simulink model "models_lib"  (R2016a)
settings: Solver=FixedStepAuto  StartTime=0.0  StopTime=30  FixedStep=0.005  RelTol=1e-3
settings Model: Creator=Shinelon  LastModifiedBy=Shinelon

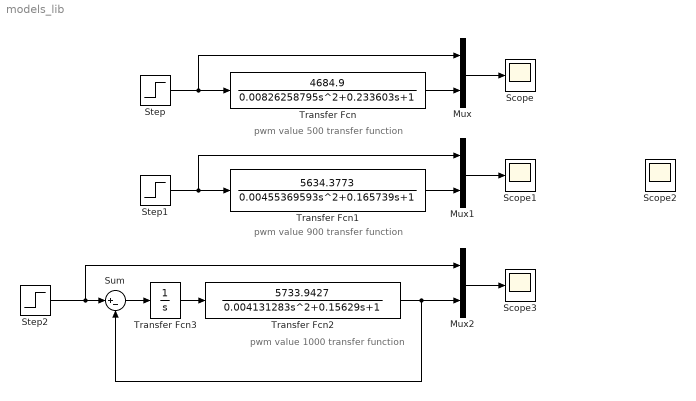
== system models_lib ==
  note: pwm value 500 transfer function
  note: pwm value 1000 transfer function
  note: pwm value 900 transfer function
  Mux : Mux  Inputs=2
  Mux1 : Mux  Inputs=2
  Mux2 : Mux  Inputs=2
  Scope{,1..3} (4 alike) : Scope
  Step : Step  Time=0.11  After=4.139  SampleTime=0.005
  Step1 : Step  Time=0.11  After=11.59*900/1400  SampleTime=0.005
  Step2 : Step  Time=0.11  After=4.139  SampleTime=0.005
  Sum : Sum  Inputs=|+-
  Transfer Fcn : TransferFcn  Numerator=[4684.9]  Denominator="[0.00826258795  0.233603 1]"
  Transfer Fcn1 : TransferFcn  Numerator=[5634.3773]  Denominator="[0.00455369593  0.165739 1]"
  Transfer Fcn2 : TransferFcn  Numerator=[5733.9427]  Denominator="[0.004131283  0.15629 1]"
  Transfer Fcn3 : TransferFcn  Denominator=[1 0]
  wires:
  Step/1 -> Transfer Fcn/1, Mux/1
  Mux/1 -> Scope/1
  Transfer Fcn/1 -> Mux/2
  Mux2/1 -> Scope3/1
  Transfer Fcn2/1 -> Sum/2, Mux2/2
  Step1/1 -> Transfer Fcn1/1, Mux1/1
  Mux1/1 -> Scope1/1
  Transfer Fcn1/1 -> Mux1/2
  Step2/1 -> Mux2/1, Sum/1
  Sum/1 -> Transfer Fcn3/1
  Transfer Fcn3/1 -> Transfer Fcn2/1
